simulink model "lowpassdisc"  (Simulink 8.3)
settings: Solver=FixedStepDiscrete  StartTime=0.0  StopTime=10.24  FixedStep=dt  MaxStep=自動  MinStep=自動  RelTol=1e-3  AbsTol=自動
values from neighbouring files (symbols this model uses):
  dt = 0.01    [p217.m]    (also in p218_2.m; p223.m)
undefined symbols (not defined in the file or in its folder): den, num
settings Model: Creator=ikko  LastModifiedBy=ikko
settings SolverCC: InitialStep=自動
settings DataIOCC: SignalLoggingName=logsOut
settings OptimizationCC: ExpressionDepthLimit=2147483647  InitFltsAndDblsToZero=on
settings DebuggingCC: SaveWithParameterizedLinksMsg=none  CheckExecutionContextPreStartOutputMsg=on  CheckExecutionContextRuntimeOutputMsg=on  SignalResolutionControl=TryResolveAllWithWarning  MultiTaskDSMMsg=warning  MultiTaskCondExecSysMsg=none  FcnCallInpInsideContextMsg=EnableAllAsWarning
settings RTWCC: IncludeERTFirstTime=on
settings GRTTargetCC: TargetFcnLib=ansi_tfl_tmw.mat

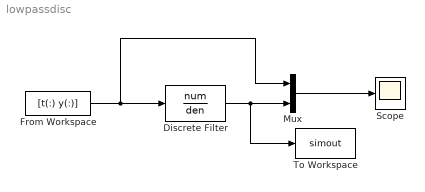
== system lowpassdisc ==
  Discrete Filter : DiscreteFilter  Numerator=num  Denominator=den
  From Workspace : FromWorkspace  VariableName=[t(:) y(:)]  SampleTime=dt
  Mux : Mux  Inputs=2
  Scope : Scope
  To Workspace : ToWorkspace  VariableName=simout  SaveFormat=Structure  SampleTime=-1
      settings: MaxDataPoints=length(t)
  wires:
  Discrete Filter/1 -> Mux/2, To Workspace/1
  Mux/1 -> Scope/1
  From Workspace/1 -> Mux/1, Discrete Filter/1
